simulink subsystem "Sub_Encoders_Piero6"  (R2023b)
settings: Solver=VariableStepAuto  StartTime=0.0  StopTime=10.0  RelTol=1e-3
libraries: simulink x1
settings Model: Creator=Usuario  LastModifiedBy=Usuario

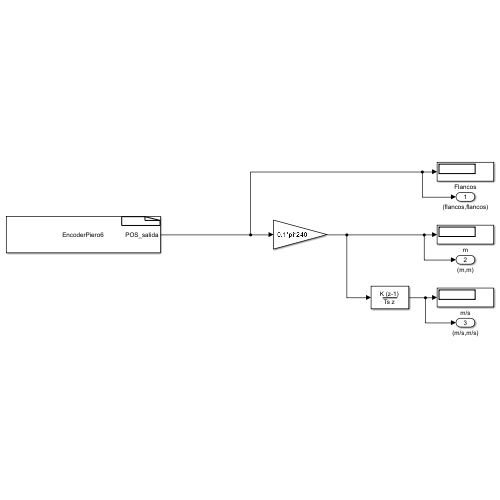
[thumbnail: Simulink's stored preview of the top-level diagram]
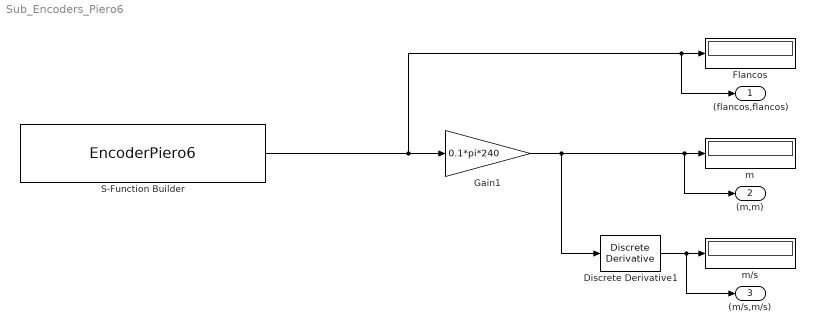
== system Sub_Encoders_Piero6 ==
  Discrete Derivative1 : simulink/Discrete/Discrete Derivative  gainval=1.0  ICPrevScaledInput=0.0  OutMin=[]  OutMax=[]  OutDataType=fixdt(1, 16)  OutScaling=2^-10  DoSatur=off
  Flancos : Display
  Gain1 : Gain  Gain=0.1*pi*240
  S-Function Builder : S-Function  FunctionName=EncoderPiero6  SFunctionModules=EncoderPiero6_wrapper.c  SFunctionDeploymentMode=off  EnableBusSupport=off  mask(S-Function Builder){}
      mask help: Simulink:masks:SFunctionBuilder_MD
      mask init:
      | val = [[.9  0.75 0.75 1 1 .9 .9 1]',[1 1 0.75 0.75 .9 .9 1 .9]'];try , sys = get_param(gcb,'SfunBuilderFcnName');if isempty(sys), sys = get_param(gcb,'FunctionName'); end,catch, sys = get_param(gcb,'FunctionName'); end
      settings: CopyFcn=set_param(gcbh,'LinkStatus','none')  OpenFcn=sfunctionwizard(gcbh)
      mask Display:
      | plot(val(:,1),val(:,2))
      | disp(sys)
      | port_label('output',1,'POS_salida')
  m : Display
  m/s : Display
  (flancos,flancos) : Outport
  (m,m) : Outport  Port=2
  (m/s,m/s) : Outport  Port=3
  wires:
  Gain1/1 -> Discrete Derivative1/1, (m,m)/1, m/1
  Discrete Derivative1/1 -> (m/s,m/s)/1, m/s/1
  S-Function Builder/1 -> Gain1/1, (flancos,flancos)/1, Flancos/1
